simulink model "Cosmin_Sim_localization"  (R2024b)
settings: Solver=VariableStepAuto  StartTime=0.0  StopTime=total_time  MaxStep=0.001  RelTol=1e-3
values from neighbouring files (symbols this model uses):
  T_s = 0.04    [EX_opt_2.m]
undefined symbols (not defined in the file or in its folder): D, d, d_used, mode, omega_trj, P_INIT_EKF, PHI_INIT, prob_gps_loss, Q_INIT, Q_INIT_LOC, r, R, R_2, R_3, R_4, R_5, r_used, total_time, Z_INIT_EKF, zoh_activation
libraries: dspsigops x2
settings Model: Creator=alberto  LastModifiedBy=cosmi
settings RTWCC: GPUComputeCapability=3.5

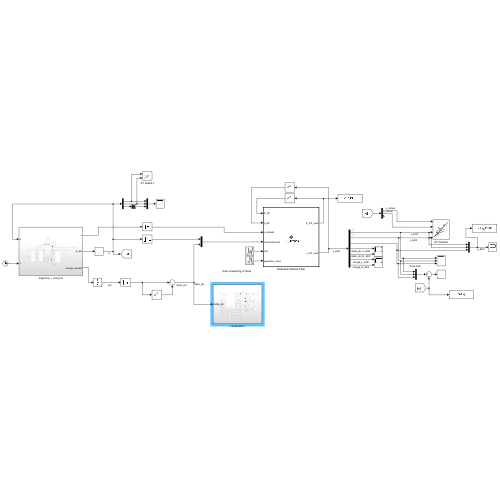
[thumbnail: Simulink's stored preview of the top-level diagram]
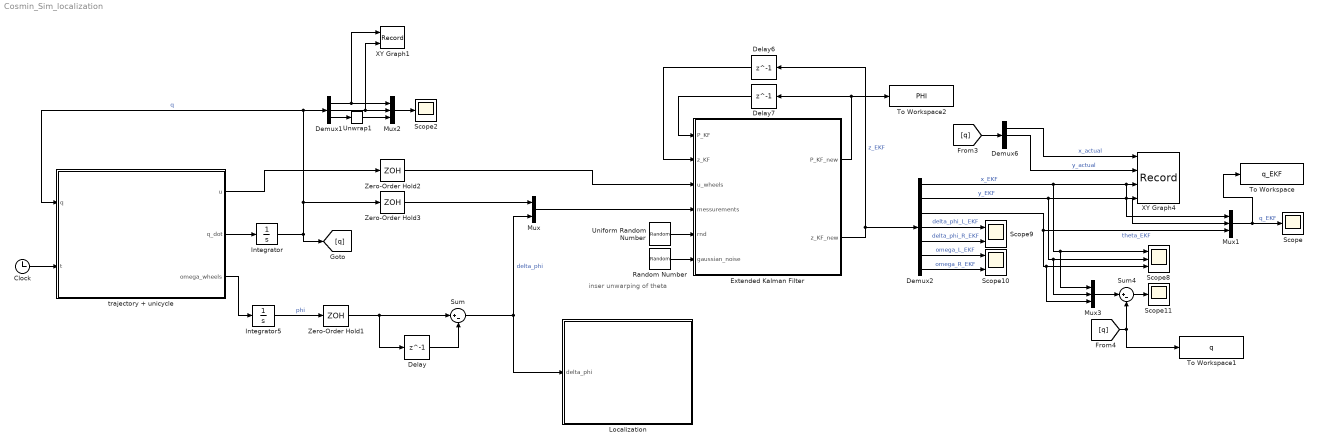
== system Cosmin_Sim_localization ==
  note: inser unwarping of theta
  Clock : Clock
  Delay : Delay  DelayLength=1  InitialCondition=[0;0]  SampleTime=T_s
  Delay6 : Delay  DelayLength=1  InitialCondition=Z_INIT_EKF  SampleTime=T_s
  Delay7 : Delay  DelayLength=1  InitialCondition=P_INIT_EKF  SampleTime=T_s
  Demux1 : Demux  Outputs=3
  Demux2 : Demux  Outputs=7
  Demux6 : Demux  Outputs=3
  Extended Kalman Filter : MATLAB Function  TreatAsAtomicUnit=on
  Integrator : Integrator  InitialCondition=Q_INIT
  Integrator5 : Integrator  InitialCondition=PHI_INIT
  Localization : Subsystem
  Mux : Mux  Inputs=2
  Mux1 : Mux  Inputs=3
  Mux2 : Mux  Inputs=3
  Mux3 : Mux  Inputs=3
  Random Number : RandomNumber  Variance=0.00001  SampleTime=T_s
  Scope : Scope
  Scope10 : Scope  NumInputPorts=2
  Scope11 : Scope
  Scope2 : Scope
  Scope8 : Scope  NumInputPorts=3
  Scope9 : Scope  NumInputPorts=2
  Sum : Sum  Inputs=|+-
  Sum4 : Sum  Inputs=|+-
  To Workspace : ToWorkspace  VariableName=q_EKF  SampleTime=-1
  To Workspace1 : ToWorkspace  VariableName=q  SampleTime=-1
  To Workspace2 : ToWorkspace  VariableName=PHI  SampleTime=-1
  Uniform Random Number : UniformRandomNumber  Minimum=0  SampleTime=T_s
  Unwrap1 : dspsigops/Unwrap  tol=pi  InputProcessing=Columns as channels (frame based)  running=off
  XY Graph1 : Record  FileSettingsInternal="{\"entries\":[{\"content\":{\"excelSettings\":{\"content\":{},\"type\":\"Streamout.ExcelSettings\"}},\"type\":\"Streamout.FileSettingStorage\",\"uuid\":\"\"}],\"packageUris\":[\"http:\\/\\/schema.mathworks.com\\/mf0\\/streamout_blocks\\/R2020a\"],\"version\":\"1.0\"}"  Layout=[1 1]  SignalsInternal="{\"entries\":[{\"content\":{\"signals\":[{\"content\":{\"blockPath\":[],\"dimensions\":[1,1],\"domain\":\"\",\"lineColor\":\"#a2142f\",\"lineWidth\":2,\"port\":1,\"sid\":[\"\"],\"signalID\":1,\"signalName\":\"Demux1:1\"},\"type\":\"RecordBlkView.Signal\",\"uuid\":\"\"},{\"content\":{\"blockPath\":[],\"dimensions\":[1,1],\"domain\":\"\",\"lineColor\":\"#139fff\",\"lineWidth\":2,\"port\":2,\"sid\":[\"\"],\"signalID\":2,\"signalName\":\"Demux1:2\"},\"type\":\"RecordBlkView.Signal\",\"uuid\":\"\"}]},\"type\":\"RecordBlkView.InputSignals\",\"uuid\":\"\"}],\"packageUris\":[\"http:\\/\\/schema.mathworks.com\\/mf0\\/streamout_blocks\\/R2020a\"],\"version\":\"1.0\"}"  VisualizationBindings="{\"xyplotplugin\":{\"info\":[{\"series\":[],\"subplotID\":1}]}}"  CompatibilityTag=XY
  XY Graph4 : Record  FileSettingsInternal="{\"entries\":[{\"content\":{\"excelSettings\":{\"content\":{},\"type\":\"Streamout.ExcelSettings\"}},\"type\":\"Streamout.FileSettingStorage\",\"uuid\":\"\"}],\"packageUris\":[\"http:\\/\\/schema.mathworks.com\\/mf0\\/streamout_blocks\\/R2020a\"],\"version\":\"1.0\"}"  Layout=[1 1]  SignalsInternal="{\"entries\":[{\"content\":{\"signals\":[{\"content\":{\"blockPath\":[],\"dimensions\":[1,1],\"domain\":\"\",\"lineColor\":\"#ff6929\",\"lineWidth\":2,\"port\":1,\"sid\":[\"\"],\"signalID\":1,\"signalName\":\"x_actual\"},\"type\":\"RecordBlkView.Signal\",\"uuid\":\"\"},{\"content\":{\"blockPath\":[],\"dimensions\":[1,1],\"domain\":\"\",\"lineColor\":\"#b746ff\",\"lineWidth\":2,\"port\":2,\"sid\":[\"\"],\"signalID\":2,\"signalName\":\"y_actual\"},\"type\":\"RecordBlkView.Signal\",\"uuid\":\"\"},{\"content\":{\"blockPath\":[],\"dimensions\":[1,1],\"domain\":\"\",\"lineColor\":\"#64d413\",\"lineWidth\":2,\"plots\":[ 1 ],\"port\":3,\"sid\":[\"\"],\"signalID\":3,\"signalName\":\"x_EKF\"},\"type\":\"RecordBlkView.Signal\",\"uuid\":\"\"},{\"content\":{\"blockPath\":[],\"dimensions\":[1,1],\"domain\":\"\",\"lineColor\":\"#ff13a6\",\"lineWidth\":2,\"plots\":[ 1 ],\"port\":4,\"sid\":[\"\"],\"signalID\":4,\"signalName\":\"y_EKF\"},\"type\":\"RecordBlkView.Signal\",\"uuid\":\"\"}]},\"type\":\"RecordBlkView.InputSignals\",\"uuid\":\"\"}],\"packageUris\":[\"http:\\/\\/schema.mathworks.com\\/mf0\\/streamout_blocks\\/R2020a\"],\"version\":\"1.0\"}"  VisualizationBindings="{\"xyplotplugin\":{\"info\":[{\"series\":[{\"bindingParametersList\":[{\"parameter\":\"X-Axis\",\"signalID\":3,\"signalName\":\"x_EKF\"},{\"parameter\":\"Y-Axis\",\"signalID\":4,\"signalName\":\"y_EKF\"},{\"parameter\":\"X-Axis\",\"signalID\":3,\"signalName\":\"x_EKF\"},{\"parameter\":\"Y-Axis\",\"signalID\":4,\"signalName\":\"y_EKF\"}],\"seriesID\":0}],\"subplotID\":1}]}}"  CompatibilityTag=XY
  Zero-Order Hold1 : ZeroOrderHold  SampleTime=T_s
  Zero-Order Hold2 : ZeroOrderHold  SampleTime=T_s
  Zero-Order Hold3 : ZeroOrderHold  SampleTime=T_s
  trajectory + unicycle : Subsystem
  wires:
  Zero-Order Hold1/1 -> Sum/1, Delay/1
  Delay/1 -> Sum/2
  Integrator/1 -> [q], trajectory + unicycle/1(q), Demux1/1, Zero-Order Hold3/1  "q"
  Integrator5/1 -> Zero-Order Hold1/1  "phi"
  Unwrap1/1 -> Mux2/3
  Demux1/3 -> Unwrap1/1
  Demux1/2 -> XY Graph1/2, Mux2/2
  Demux1/1 -> XY Graph1/1, Mux2/1
  Mux2/1 -> Scope2/1
  Zero-Order Hold3/1 -> Mux/1
  Sum/1 -> Localization/1(delta_phi), Mux/2  "delta_phi"
  Demux2/1 -> Mux3/1, Scope8/1, Mux1/1, XY Graph4/3  "x_EKF"
  Zero-Order Hold2/1 -> Extended Kalman Filter/3(u_wheels)
  Mux/1 -> Extended Kalman Filter/4(messurements)
  Delay6/1 -> Extended Kalman Filter/2(z_KF)
  Demux2/4 -> Scope9/1  "delta_phi_L_EKF"
  Demux2/2 -> Mux3/2, Scope8/2, Mux1/2, XY Graph4/4  "y_EKF"
  Random Number/1 -> Extended Kalman Filter/6(gaussian_noise)
  Demux6/1 -> XY Graph4/1  "x_actual"
  Demux2/6 -> Scope10/1  "omega_L_EKF"
  Delay7/1 -> Extended Kalman Filter/1(P_KF)
  Uniform Random Number/1 -> Extended Kalman Filter/5(rnd)
  Extended Kalman Filter/1(P_KF_new) -> To Workspace2/1, Delay7/1
  Demux2/3 -> Mux1/3, Mux3/3, Scope8/3  "theta_EKF"
  Demux6/2 -> XY Graph4/2  "y_actual"
  Demux2/5 -> Scope9/2  "delta_phi_R_EKF"
  Demux2/7 -> Scope10/2  "omega_R_EKF"
  Extended Kalman Filter/2(z_KF_new) -> Demux2/1, Delay6/1  "z_EKF"
  [q] -> Demux6/1
  Mux3/1 -> Sum4/1
  [q] -> To Workspace1/1, Sum4/2
  Sum4/1 -> Scope11/1
  Clock/1 -> trajectory + unicycle/2(t)
  trajectory + unicycle/1(u) -> Zero-Order Hold2/1
  trajectory + unicycle/2(q_dot) -> Integrator/1
  trajectory + unicycle/3(omega_wheels) -> Integrator5/1
  Mux1/1 -> To Workspace/1, Scope/1  "q_EKF"

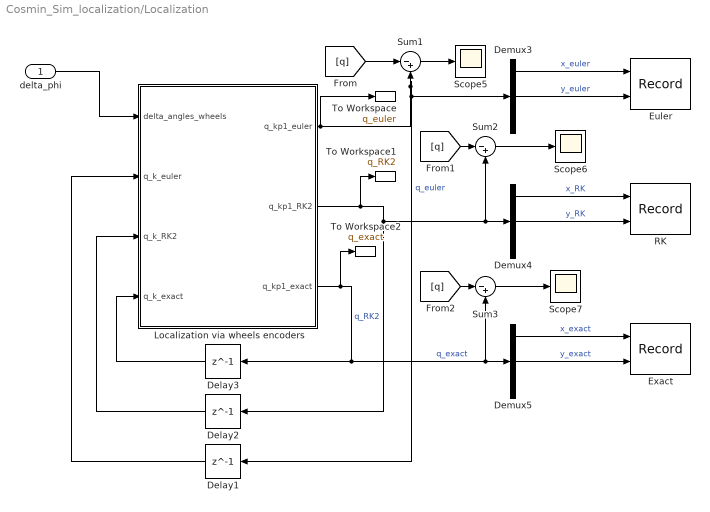
== system Cosmin_Sim_localization/Localization ==
  delta_phi : Inport
  Delay1 : Delay  DelayLength=1  InitialCondition=Q_INIT_LOC
  Delay2 : Delay  DelayLength=1  InitialCondition=Q_INIT_LOC
  Delay3 : Delay  DelayLength=1  InitialCondition=Q_INIT_LOC
  Demux3 : Demux  Outputs=3
  Demux4 : Demux  Outputs=3
  Demux5 : Demux  Outputs=3
  Euler : Record  FileSettingsInternal="{\"entries\":[{\"content\":{\"excelSettings\":{\"content\":{},\"type\":\"Streamout.ExcelSettings\"}},\"type\":\"Streamout.FileSettingStorage\",\"uuid\":\"\"}],\"packageUris\":[\"http:\\/\\/schema.mathworks.com\\/mf0\\/streamout_blocks\\/R2020a\"],\"version\":\"1.0\"}"  Layout=[1 1]  SignalsInternal="{\"entries\":[{\"content\":{\"signals\":[{\"content\":{\"blockPath\":[],\"dimensions\":[1,1],\"domain\":\"\",\"lineColor\":\"#edb120\",\"lineWidth\":2,\"port\":1,\"sid\":[\"\"],\"signalID\":1,\"signalName\":\"x_euler\"},\"type\":\"RecordBlkView.Signal\",\"uuid\":\"\"},{\"content\":{\"blockPath\":[],\"dimensions\":[1,1],\"domain\":\"\",\"lineColor\":\"#7e2f8e\",\"lineWidth\":2,\"port\":2,\"sid\":[\"\"],\"signalID\":2,\"signalName\":\"y_euler\"},\"type\":\"RecordBlkView.Signal\",\"uuid\":\"\"}]},\"type\":\"RecordBlkView.InputSignals\",\"uuid\":\"\"}],\"packageUris\":[\"http:\\/\\/schema.mathworks.com\\/mf0\\/streamout_blocks\\/R2020a\"],\"version\":\"1.0\"}"  VisualizationBindings="{\"xyplotplugin\":{\"info\":[{\"series\":[],\"subplotID\":1}]}}"  CompatibilityTag=XY
  Exact : Record  FileSettingsInternal="{\"entries\":[{\"content\":{\"excelSettings\":{\"content\":{},\"type\":\"Streamout.ExcelSettings\"}},\"type\":\"Streamout.FileSettingStorage\",\"uuid\":\"\"}],\"packageUris\":[\"http:\\/\\/schema.mathworks.com\\/mf0\\/streamout_blocks\\/R2020a\"],\"version\":\"1.0\"}"  Layout=[1 1]  SignalsInternal="{\"entries\":[{\"content\":{\"signals\":[{\"content\":{\"blockPath\":[],\"dimensions\":[1,1],\"domain\":\"\",\"lineColor\":\"#77ac30\",\"lineWidth\":2,\"port\":1,\"sid\":[\"\"],\"signalID\":1,\"signalName\":\"x_exact\"},\"type\":\"RecordBlkView.Signal\",\"uuid\":\"\"},{\"content\":{\"blockPath\":[],\"dimensions\":[1,1],\"domain\":\"\",\"lineColor\":\"#4dbeee\",\"lineWidth\":2,\"port\":2,\"sid\":[\"\"],\"signalID\":2,\"signalName\":\"y_exact\"},\"type\":\"RecordBlkView.Signal\",\"uuid\":\"\"}]},\"type\":\"RecordBlkView.InputSignals\",\"uuid\":\"\"}],\"packageUris\":[\"http:\\/\\/schema.mathworks.com\\/mf0\\/streamout_blocks\\/R2020a\"],\"version\":\"1.0\"}"  VisualizationBindings="{\"xyplotplugin\":{\"info\":[{\"series\":[],\"subplotID\":1}]}}"  CompatibilityTag=XY
  Localization via wheels encoders : MATLAB Function  TreatAsAtomicUnit=on
  RK : Record  FileSettingsInternal="{\"entries\":[{\"content\":{\"excelSettings\":{\"content\":{},\"type\":\"Streamout.ExcelSettings\"}},\"type\":\"Streamout.FileSettingStorage\",\"uuid\":\"\"}],\"packageUris\":[\"http:\\/\\/schema.mathworks.com\\/mf0\\/streamout_blocks\\/R2020a\"],\"version\":\"1.0\"}"  Layout=[1 1]  SignalsInternal="{\"entries\":[{\"content\":{\"signals\":[{\"content\":{\"blockPath\":[],\"dimensions\":[1,1],\"domain\":\"\",\"lineColor\":\"#a2142f\",\"lineWidth\":2,\"plots\":[ 1 ],\"port\":1,\"sid\":[\"\"],\"signalID\":1,\"signalName\":\"x_RK\"},\"type\":\"RecordBlkView.Signal\",\"uuid\":\"\"},{\"content\":{\"blockPath\":[],\"dimensions\":[1,1],\"domain\":\"\",\"lineColor\":\"#139fff\",\"lineWidth\":2,\"plots\":[ 1 ],\"port\":2,\"sid\":[\"\"],\"signalID\":2,\"signalName\":\"y_RK\"},\"type\":\"RecordBlkView.Signal\",\"uuid\":\"\"}]},\"type\":\"RecordBlkView.InputSignals\",\"uuid\":\"\"}],\"packageUris\":[\"http:\\/\\/schema.mathworks.com\\/mf0\\/streamout_blocks\\/R2020a\"],\"version\":\"1.0\"}"  VisualizationBindings="{\"xyplotplugin\":{\"info\":[{\"series\":[{\"bindingParametersList\":[{\"parameter\":\"X-Axis\",\"signalID\":1,\"signalName\":\"x_RK\"},{\"parameter\":\"Y-Axis\",\"signalID\":2,\"signalName\":\"y_RK\"}],\"seriesID\":0}],\"subplotID\":1}]}}"  CompatibilityTag=XY
  Scope5 : Scope
  Scope6 : Scope
  Scope7 : Scope
  Sum1 : Sum  Inputs=|-+
  Sum2 : Sum  Inputs=|-+
  Sum3 : Sum  Inputs=|-+
  To Workspace : ToWorkspace  VariableName=q_euler  SampleTime=-1
  To Workspace1 : ToWorkspace  VariableName=q_RK2  SampleTime=-1
  To Workspace2 : ToWorkspace  VariableName=q_exact  SampleTime=-1
  wires:
  delta_phi/1 -> Localization via wheels encoders/1(delta_angles_wheels)
  Localization via wheels encoders/1(q_kp1_euler) -> Demux3/1, Delay1/1, Sum1/2, To Workspace/1  "q_euler"
  [q] -> Sum3/1
  Demux3/2 -> Euler/2  "y_euler"
  Localization via wheels encoders/2(q_kp1_RK2) -> To Workspace1/1, Sum2/2, Demux4/1, Delay2/1  "q_RK2"
  [q] -> Sum1/1
  Demux4/2 -> RK/2  "y_RK"
  Demux3/1 -> Euler/1  "x_euler"
  Sum3/1 -> Scope7/1
  Demux5/1 -> Exact/1  "x_exact"
  Demux5/2 -> Exact/2  "y_exact"
  Sum1/1 -> Scope5/1
  Delay3/1 -> Localization via wheels encoders/4(q_k_exact)
  Delay1/1 -> Localization via wheels encoders/2(q_k_euler)
  Localization via wheels encoders/3(q_kp1_exact) -> To Workspace2/1, Delay3/1, Demux5/1, Sum3/2  "q_exact"
  [q] -> Sum2/1
  Demux4/1 -> RK/1  "x_RK"
  Delay2/1 -> Localization via wheels encoders/3(q_k_RK2)
  Sum2/1 -> Scope6/1

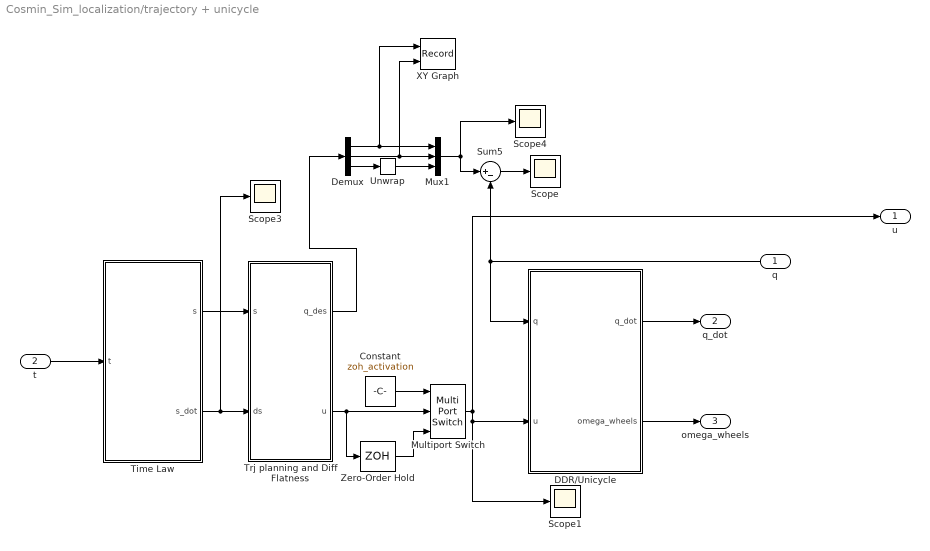
== system Cosmin_Sim_localization/trajectory + unicycle ==
  q : Inport
  t : Inport  Port=2
  Constant : Constant  Value=zoh_activation
  DDR/Unicycle : MATLAB Function  TreatAsAtomicUnit=on
  Demux : Demux  Outputs=3
  Multiport Switch : MultiPortSwitch  Inputs=2  SaturateOnIntegerOverflow=off  InputSameDT=off
  Mux1 : Mux  Inputs=3
  Scope{,1,3..4} (4 alike) : Scope
  Sum5 : Sum  Inputs=|+-
  Time Law : MATLAB Function  TreatAsAtomicUnit=on
  Trj planning and Diff Flatness : MATLAB Function  TreatAsAtomicUnit=on
  Unwrap : dspsigops/Unwrap  tol=pi  InputProcessing=Columns as channels (frame based)  running=off
  XY Graph : Record  FileSettingsInternal="{\"entries\":[{\"content\":{\"excelSettings\":{\"content\":{},\"type\":\"Streamout.ExcelSettings\"}},\"type\":\"Streamout.FileSettingStorage\",\"uuid\":\"\"}],\"packageUris\":[\"http:\\/\\/schema.mathworks.com\\/mf0\\/streamout_blocks\\/R2020a\"],\"version\":\"1.0\"}"  Layout=[1 1]  SignalsInternal="{\"entries\":[{\"content\":{\"signals\":[{\"content\":{\"blockPath\":[],\"dimensions\":[1,1],\"domain\":\"\",\"lineColor\":\"#77ac30\",\"lineWidth\":2,\"port\":1,\"sid\":[\"\"],\"signalID\":1,\"signalName\":\"Demux:1\"},\"type\":\"RecordBlkView.Signal\",\"uuid\":\"\"},{\"content\":{\"blockPath\":[],\"dimensions\":[1,1],\"domain\":\"\",\"lineColor\":\"#4dbeee\",\"lineWidth\":2,\"port\":2,\"sid\":[\"\"],\"signalID\":2,\"signalName\":\"Demux:2\"},\"type\":\"RecordBlkView.Signal\",\"uuid\":\"\"}]},\"type\":\"RecordBlkView.InputSignals\",\"uuid\":\"\"}],\"packageUris\":[\"http:\\/\\/schema.mathworks.com\\/mf0\\/streamout_blocks\\/R2020a\"],\"version\":\"1.0\"}"  VisualizationBindings="{\"xyplotplugin\":{\"info\":[{\"series\":[],\"subplotID\":1}]}}"  CompatibilityTag=XY
  Zero-Order Hold : ZeroOrderHold  SampleTime=T_s
  u : Outport
  q_dot : Outport  Port=2
  omega_wheels : Outport  Port=3
  wires:
  q/1 -> Sum5/2, DDR/Unicycle/1(q)
  Demux/2 -> XY Graph/2, Mux1/2
  Time Law/1(s) -> Trj planning and Diff Flatness/1(s)
  Constant/1 -> Multiport Switch/1
  Mux1/1 -> Sum5/1, Scope4/1
  Trj planning and Diff Flatness/2(u) -> Zero-Order Hold/1, Multiport Switch/2
  Multiport Switch/1 -> u/1, Scope1/1, DDR/Unicycle/2(u)
  Time Law/2(s_dot) -> Scope3/1, Trj planning and Diff Flatness/2(ds)
  Demux/1 -> XY Graph/1, Mux1/1
  Sum5/1 -> Scope/1
  Demux/3 -> Unwrap/1
  Unwrap/1 -> Mux1/3
  DDR/Unicycle/2(omega_wheels) -> omega_wheels/1
  Zero-Order Hold/1 -> Multiport Switch/3
  Trj planning and Diff Flatness/1(q_des) -> Demux/1
  DDR/Unicycle/1(q_dot) -> q_dot/1
  t/1 -> Time Law/1(t)

== matlab function Cosmin_Sim_localization/trajectory + unicycle/Time Law ==
  data: t input; s output; s_dot output; total_time parameter; mode parameter
function [s, s_dot] = fcn(t,total_time, mode)
s=0;
s_dot=0;
if mode==1%if mode =1 costasnt time law else trapezoidal
    s_dot = 1/total_time;
    s=t/total_time;
else
    Ta=0.5;% acceleration/dec time 10% of total
    Tc=9;%time of costant time

    Vc=1/(Ta+Tc);% velocità costante
    a=Vc/Ta;% acceleration
    
    switch 1 %formula on the slide
        case t<Ta
            s_dot=a*t;
            s=(a*(t^2))/2;

        case (t>=Ta)&&(t<(Tc+Ta))
            s_dot=Vc;
            s=(a*(Ta^2))/2+Vc*(t-Ta);

        case (t>=(Tc+Ta))&&(t<(Tc+2*Ta))
            s_dot=Vc-a*(t-Ta-Tc);
            s=(a*(Ta^2))/2+Vc*Tc+Vc*(t-Ta-Tc)-a*(t-Ta-Tc)^2/2;

        case t>=(Tc+2*Ta)
            s_dot=0;
            s=1;
    end

end

== matlab function Cosmin_Sim_localization/trajectory + unicycle/DDR//Unicycle ==
  data: q input; u input; q_dot output; omega_wheels output; d_used parameter; r_used parameter
function [q_dot, omega_wheels] = DDR_Unicycle(q, u, d_used, r_used)
v = u(1);
omega = u(2);

q_dot = [cos(q(3))*v; sin(q(3))*v; omega];

%evaluation of speed wheels
omega_L = (v - d_used*omega) / (2*r_used);
omega_R = (v + d_used*omega) / (2*r_used);
omega_wheels=[omega_R; omega_L];

== matlab function Cosmin_Sim_localization/trajectory + unicycle/Trj planning and Diff Flatness ==
  data: q_des output; s input; u output; ds input; R parameter; omega_trj parameter
function [q_des, u] = get_inputs(s, ds,R,omega_trj)

x=R*sin(2*omega_trj.*s);
y=R*sin(omega_trj.*s);

x_dot = R*2*omega_trj*cos(2*omega_trj.*s);
y_dot = R*omega_trj*cos(omega_trj.*s);

x_ddot = R*4*omega_trj*omega_trj*(-sin(2*omega_trj.*s));
y_ddot = R*omega_trj*omega_trj*(-sin(omega_trj.*s));

theta = atan2(y_dot,x_dot);

%   v
v = ds.*sqrt(y_dot.^2 + x_dot.^2);

%   omega
w = ds.*(x_dot.*y_ddot - y_dot.*x_ddot)./(y_dot.^2 + x_dot.^2);
    
q_des = [x; y; theta];
u = [v; w];

== matlab function Cosmin_Sim_localization/Localization/Localization via wheels encoders ==
  data: delta_angles_wheels input; q_k_euler input; q_k_RK2 input; q_k_exact input; r parameter; d parameter; q_kp1_euler output; T_s parameter; q_kp1_RK2 output; q_kp1_exact output
function [q_kp1_euler, q_kp1_RK2, q_kp1_exact] = localization(delta_angles_wheels, q_k_euler, q_k_RK2, q_k_exact, r, d, T_s)

    v_k = r * (delta_angles_wheels(2) + delta_angles_wheels(1)) / (T_s * 2);
    w_k = r * (delta_angles_wheels(1) - delta_angles_wheels(2)) / (T_s * d);
    
    % Euler integration
    x_kp1_euler     = q_k_euler(1) + T_s * v_k * cos(q_k_euler(3));
    y_kp1_euler     = q_k_euler(2) + T_s * v_k * sin(q_k_euler(3));
    theta_kp1_euler = q_k_euler(3) + T_s * w_k;
    q_kp1_euler     = [x_kp1_euler; y_kp1_euler; theta_kp1_euler];
    
    % Runge-Kutta 2
    x_kp1_RK2       = q_k_RK2(1) + T_s * v_k * cos(q_k_RK2(3) + T_s * w_k / 2);
    y_kp1_RK2       = q_k_RK2(2) + T_s * v_k * sin(q_k_RK2(3) + T_s * w_k / 2);
    theta_kp1_RK2   = q_k_RK2(3) + T_s * w_k;
    q_kp1_RK2       = [x_kp1_RK2; y_kp1_RK2; theta_kp1_RK2];
    
    % Exact Integration
    x_kp1_exact     = q_k_exact(1) + (v_k / w_k) * (sin(q_k_exact(3) + w_k*T_s) - sin(q_k_exact(3)));
    y_kp1_exact     = q_k_exact(2) - (v_k / w_k) * (cos(q_k_exact(3) + w_k*T_s) - cos(q_k_exact(3)));
    theta_kp1_exact = q_k_exact(3) + T_s * w_k;
    
    % The problem with Exact integration fixed by switching strategy
    if abs(delta_angles_wheels(2) - delta_angles_wheels(1)) <= 0.001
        q_kp1_exact = [x_kp1_RK2; y_kp1_RK2; theta_kp1_RK2];
    else
        q_kp1_exact = [x_kp1_exact; y_kp1_exact; theta_kp1_exact];
    end

end

== matlab function Cosmin_Sim_localization/Extended Kalman Filter ==
  data: P_KF input; P_KF_new output; z_KF input; z_KF_new output; u_wheels input; messurements input; D parameter; R_2 parameter; R_3 parameter; R_4 parameter; R_5 parameter; T_s parameter; r parameter; d parameter; prob_gps_loss parameter; rnd input; gaussian_noise input
function [P_KF_new, z_KF_new] = EKF_filtering(P_KF, z_KF, u_wheels, messurements, D, R_2, R_3, R_4, R_5 ,T_s, r, d, prob_gps_loss, rnd, gaussian_noise)

% z_KF = [x_EKF, y_EKF, theta_EKF, delta_phi_L_EKF, delta_phi_R_EKF, omega_L_EKF, omega_R_EKF]

v_k = r * (z_KF(6) + z_KF(7))/2;
w_k = r * (z_KF(7) - z_KF(6))/d;

theta_mean = z_KF(3) + (w_k * T_s)/2;

F_k = [1, 0, -T_s * v_k * sin(theta_mean), 0, 0, T_s * r * cos(theta_mean)/2 + (T_s)^2 * r * v_k * sin(theta_mean)/(2*d), T_s * r * cos(theta_mean)/2 - (T_s)^2 * r * v_k * sin(theta_mean)/(2*d);
    0, 1, T_s * v_k * cos(theta_mean), 0, 0, T_s * r * sin(theta_mean)/2 - (T_s)^2 * r * v_k * cos(theta_mean)/(2*d), T_s * r * sin(theta_mean)/2 + (T_s)^2 * r * v_k * cos(theta_mean)/(2*d);
    0, 0, 1, 0, 0, (-T_s*r)/d, (T_s*r)/d;
    0, 0, 0, 0, 0, T_s, 0;
    0, 0, 0, 0, 0, 0, T_s;
    0, 0, 0, 0, 0, 0, 0;
    0, 0, 0, 0, 0, 0, 0];

%% Prediction part

z_pred = [z_KF(1)+(T_s*r*(z_KF(6)+z_KF(7))/2)*cos(theta_mean + (T_s*r*(z_KF(6)+z_KF(7)))/(2*d));
    z_KF(2)+(T_s*r*(z_KF(6)+z_KF(7))/2)*sin(theta_mean + (T_s*r*(z_KF(7)-z_KF(6)))/(2*d));
    theta_mean + (T_s*r*(z_KF(7)-z_KF(6))/(2*d));
    T_s*z_KF(6);
    T_s*z_KF(7);
    u_wheels(1);
    u_wheels(2)];

P_pred = F_k * P_KF * F_k' + D;


%% Update

if(rnd<=prob_gps_loss) 

    % Just encoders
    y_messurement = [messurements(4); messurements(5)];
    H = [0, 0, 0, 1, 0, 0, 0;
        0, 0, 0, 0, 1, 0, 0];

    e = y_messurement - H * z_pred;
    K = P_pred * H' /(H * P_pred * H' + R_2);

    z_KF_new = z_pred +  K * e;
    P_KF_new = P_pred - K * H * P_pred;

else 
    % GPS(x,y) + Encoders
    y_messurement = [messurements(1)+gaussian_noise;messurements(2)+gaussian_noise; messurements(4); messurements(5)];

    H = [1, 0, 0, 0, 0, 0, 0;
         0, 1, 0, 0, 0, 0, 0;
         0, 0, 0, 1, 0, 0, 0;
         0, 0, 0, 0, 1, 0, 0];

    e = y_messurement - H * z_pred;
    K = P_pred * H' /(H * P_pred * H' + R_4);

    z_KF_new = z_pred + K * e;
    P_KF_new = P_pred - K * H * P_pred;

end
